simulink model "target_transmit_singleThreshold_MFB"  (R2015a)
settings: Solver=FixedStepDiscrete  StartTime=0  StopTime=inf  RelTol=1e-3
model workspace (MAT data in the model file):
  dt = 0.1
undefined symbols (not defined in the file or in its folder): gray, IsPositionTracked, IsSkeletonTracked, jet, JointDepthIndices, JointImageIndices, JointTrackingState, JointWorldCoordinates, none, PositionDepthIndices, PositionImageIndices, PositionWorldCoordinates, SegmentationData, SkeletonTrackingID, videoinput
libraries: visionsinks x5, visiontextngfix x3, embdlinuxlib x2, visionconversions x1, dspvision x1, imaqlib x1, sldrtlib x1
settings Model: PauseTimes=89  ExtModeTrigDuration=100  Creator=sbiagion  LastModifiedBy=sbiagion
settings DataIOCC: SaveFormat=StructureWithTime
settings OptimizationCC: OptimizeModelRefInitCode=on  LifeSpan=1
settings DebuggingCC: UnderspecifiedInitializationDetection=Classic  MergeDetectMultiDrivingBlocksExec=none
settings HardwareCC: ProdLargestAtomicInteger=Long  ProdLargestAtomicFloat=Double  ProdEndianess=LittleEndian  ProdHWDeviceType=ARM Compatible->ARM Cortex
settings RTWCC: SystemTargetFile=realtime.tlc  GenerateMakefile=off  TemplateMakefile=realtime.tmf  Description=Run on Target Hardware  RTWVerbose=off
settings STFCustomTargetCC: CodeReplacementLibrary=C89/C90 (ANSI)
settings ERTTargetCC: CodeReplacementLibrary=C89/C90 (ANSI)  CombineOutputUpdateFcns=off  ExtModeMexArgs='172.28.64.170' 0 17725  ERTSrcFileBannerTemplate=realtime_code_template.cgt  ERTHdrFileBannerTemplate=realtime_code_template.cgt  ERTDataSrcFileTemplate=realtime_code_template.cgt  ERTDataHdrFileTemplate=realtime_code_template.cgt  ERTCustomFileTemplate=realtime_file_process.tlc

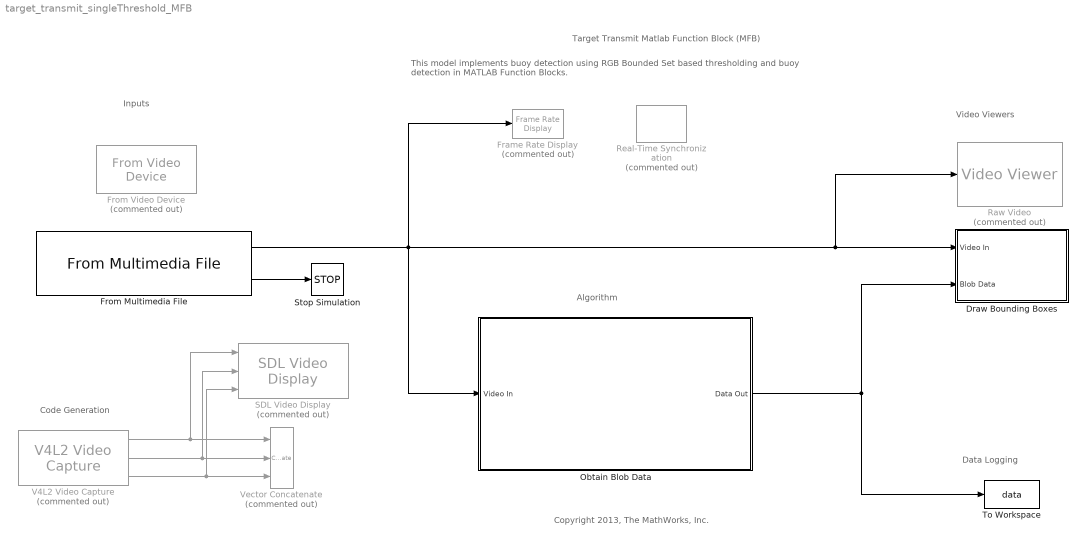
== system target_transmit_singleThreshold_MFB ==
  note: Copyright 2013, The MathWorks, Inc.
  note: Data Logging
  note: Algorithm
  note: Video Viewers
  note: Inputs
  note: Code Generation
  note: This model implements buoy detection using RGB Bounded Set based thresholding
      | and buoy detection in MATLAB Function Blocks.
  note: Target Transmit Matlab Function Block (MFB)
  Draw Bounding Boxes : Subsystem
  Frame Rate Display : visionsinks/Frame Rate Display  Commented=on  UpdateRate=10
  From Multimedia File : dspvision/From Multimedia File  inputFilename=..\..\media\rawVideo_640x480.avi  loop=on  numPlays=1  outputStreams=Video only  videoDataType=uint8  audioDataType=int16  inheritSampleTime=on  userDefinedSampleTime=0.1  noAudioOutput=off  isIntensityVideo=off  fourcc=RGB  colorVideoFormat=One multidimensional signal  outputEOF=on  dataOrg=Column-major  audioFrameSize=1024  computeAudioFrameSize=off  outSamplingMode=Sample based
  From Video Device : imaqlib/From Video Device  Commented=on  DeviceMenu=(none)  Device=winvideo 1 (Microsoft LifeCam Cinema)  ObjConstructor=videoinput('winvideo', 1)  VideoFormatMenu=(none)  VideoFormat=MJPG_640x480  VideoSource=input1  ROIPosition=[0 0 480 640]  EnableHWTrigger=off  TriggerConfiguration=none/none  SampleTime=0.1  OutputPortsMode=One multidimensional signal  DataType=single  CanDoHWTrigger=no  ReturnedColorSpace=rgb  BlockHandle=2792.0001  ROIWidth=640  ROIHeight=480  ROIColumn=0  ROIRow=0  EngXMLPath=C:\Program Files\MATLAB\R2015a\toolbox\imaq\imaq\private  DevXMLPath=C:\Program Files\MATLAB\R2015a\toolbox\imaq\imaqadaptors\win64  EngLibPath=C:\Program Files\MATLAB\R2015a\toolbox\imaq\imaqblks\imaqmex\win64  ColorSpace=rgb  BayerSensorAlignment=grbg  AllMetadata=IsPositionTracked;IsSkeletonTracked;JointDepthIndices;JointImageIndices;JointTrackingState;JointWorldCoordinates;PositionDepthIndices;PositionImageIndices;PositionWorldCoordinates;SegmentationData;SkeletonTrackingID
  Obtain Blob Data : Subsystem  VariantControl=boundedVariant
  "Raw Video " : visionsinks/Video Viewer  Commented=on  inputType=Obsolete7b  imagePorts=One multidimensional signal  useColorMap=off  colormapValue=gray(256)  specRange=off  minInputVal=0  maxInputVal=255  FigPos=[1096 875 817 565]  AxisZoom=on  trueSizedOnce=off  OpenAtMdlStart=on  DefaultConfigurationName=vipscopes.VideoViewerScopeCfg
  Real-Time Synchronization : sldrtlib/Real-Time Synchronization  Commented=on  SampleTime=0.1  MaxMissedTicks=1e9  ShowMissedTicks=off  YieldWhenWaiting=off
  SDL Video Display : embdlinuxlib/SDL Video Display  Commented=on  pixelFormat=RGB  pixelOrder=Planar  rowMajor=on  blockPlatform=BeagleBoard
  Stop Simulation : Stop
  To Workspace : ToWorkspace  VariableName=data  SaveFormat=Timeseries  SampleTime=-1
  V4L2 Video Capture : embdlinuxlib/V4L2 Video Capture  Commented=on  m_devName='/dev/video0'  roi=[0, 0, 640, 480]  imSizeSelection=640x480  imSize=[640, 480]  pixelFormat=RGB  pixelOrder=Planar  sampleTime=1/30  simOutput=Colorbars  blockPlatform=BeagleBoard
  Vector Concatenate : Concatenate  Commented=on  NumInputs=3  Mode=Multidimensional array  ConcatenateDimension=3
  wires:
  From Multimedia File/2 -> Stop Simulation/1
  V4L2 Video Capture/1 -> SDL Video Display/1, Vector Concatenate/1
  V4L2 Video Capture/2 -> SDL Video Display/2, Vector Concatenate/2
  V4L2 Video Capture/3 -> SDL Video Display/3, Vector Concatenate/3
  Obtain Blob Data/1(Data Out) -> Draw Bounding Boxes/2(Blob Data), To Workspace/1
  From Multimedia File/1 -> Obtain Blob Data/1(Video In), Frame Rate Display/1, Draw Bounding Boxes/1(Video In), "Raw Video "/1

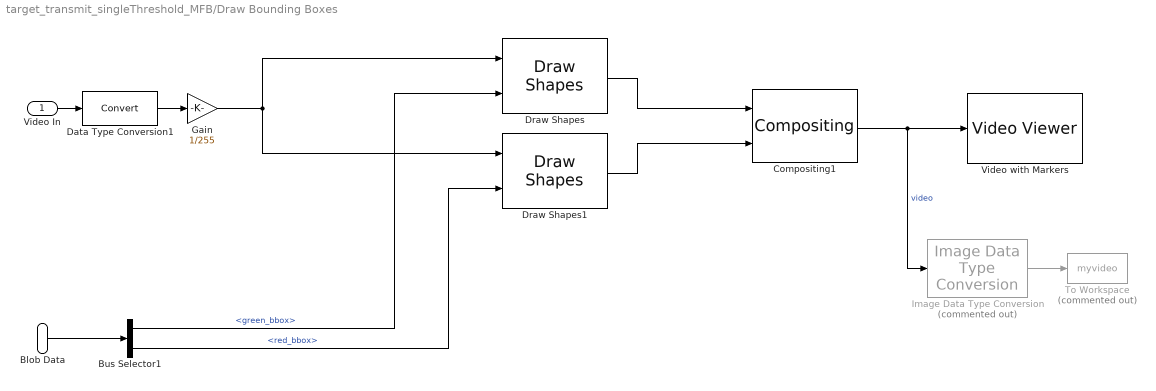
== system target_transmit_singleThreshold_MFB/Draw Bounding Boxes ==
  Video In : Inport
  Blob Data : Inport  Port=2
  Bus Selector1 : BusSelector  OutputSignals=green_bbox,red_bbox
  Compositing1 : visiontextngfix/Compositing  operation=Blend  bFacSrc=Specify via dialog  mFacSrc=Specify via dialog  bFactor=0.75  mFactor=1  source=Specify via dialog  coordinates=[1 1]  prodOutputMode=Binary point scaling  prodOutputWordLength=32  prodOutputFracLength=10  roundingMode=Floor  overflowMode=off
  Data Type Conversion1 : DataTypeConversion
  Draw Shapes : visiontextngfix/Draw Shapes  shape=Rectangles  fill=on  lineWidth=1  fillClrSource=Specify via dialog  display=User-specified value  intensity=200  color=[0 255 0]  opacity=0.5  viewport=Entire image  antialiasing=off  inType=Obsolete  imagePorts=One multidimensional signal  prodOutputMode=Binary point scaling  prodOutputWordLength=32  prodOutputFracLength=14  memoryMode=Specify word length  memoryWordLength=16  memoryFracLength=14  roundingMode=Floor  overflowMode=off
  Draw Shapes1 : visiontextngfix/Draw Shapes  shape=Rectangles  fill=on  lineWidth=1  fillClrSource=Specify via dialog  display=User-specified value  intensity=200  color=[255 0 0]  opacity=0.5  viewport=Entire image  antialiasing=off  inType=Obsolete  imagePorts=One multidimensional signal  prodOutputMode=Binary point scaling  prodOutputWordLength=32  prodOutputFracLength=14  memoryMode=Specify word length  memoryWordLength=16  memoryFracLength=14  roundingMode=Floor  overflowMode=off
  Gain : Gain  Gain=1/255
  Image Data Type Conversion : visionconversions/Image Data Type Conversion  Commented=on  outDT=uint8  isSigned=on  wordLen=16  numFracBits=0
  To Workspace : ToWorkspace  Commented=on  VariableName=myvideo  SaveFormat=Timeseries  SampleTime=-1
  Video with Markers : visionsinks/Video Viewer  inputType=Obsolete7b  imagePorts=One multidimensional signal  useColorMap=off  colormapValue=gray(256)  specRange=off  minInputVal=0  maxInputVal=255  FigPos=[791 911 843 656]  AxisZoom=on  trueSizedOnce=off  OpenAtMdlStart=on  DefaultConfigurationName=vipscopes.VideoViewerScopeCfg
  wires:
  Gain/1 -> Draw Shapes/1, Draw Shapes1/1
  Data Type Conversion1/1 -> Gain/1
  Draw Shapes1/1 -> Compositing1/2
  Draw Shapes/1 -> Compositing1/1
  Bus Selector1/1 -> Draw Shapes/2  "<green_bbox>"
  Blob Data/1 -> Bus Selector1/1
  Video In/1 -> Data Type Conversion1/1
  Compositing1/1 -> Image Data Type Conversion/1, Video with Markers/1  "video"
  Bus Selector1/2 -> Draw Shapes1/2  "<red_bbox>"
  Image Data Type Conversion/1 -> To Workspace/1

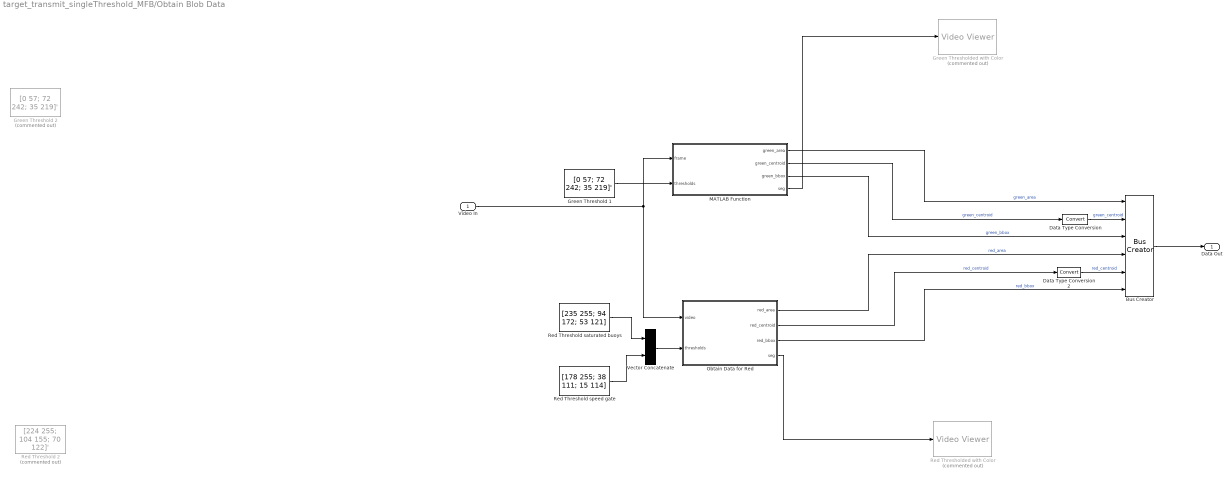
== system target_transmit_singleThreshold_MFB/Obtain Blob Data ==
  Video In : Inport
  Bus Creator : BusCreator  Inputs=6
  Data Type Conversion : DataTypeConversion
  Data Type Conversion2 : DataTypeConversion
  Green Threshold 1 : Constant  Value=[0 57; 72 242; 35 219]'  OutDataTypeStr=uint8
  Green Threshold 2 : Constant  Commented=on  Value=[0 57; 72 242; 35 219]'  OutDataTypeStr=uint8
  Green Thresholded with Color : visionsinks/Video Viewer  Commented=on  inputType=Obsolete7b  imagePorts=One multidimensional signal  useColorMap=off  colormapValue=gray(256)  specRange=off  minInputVal=0  maxInputVal=255  FigPos=[531 770 672 453]  AxisZoom=on  trueSizedOnce=off  OpenAtMdlStart=on  DefaultConfigurationName=vipscopes.VideoViewerScopeCfg
  MATLAB Function : MATLAB Function  TreatAsAtomicUnit=on
  Obtain Data for Red : MATLAB Function  TreatAsAtomicUnit=on
  Red Threshold 2 : Constant  Commented=on  Value=[224 255; 104 155; 70 122]'  OutDataTypeStr=uint8
  Red Threshold saturated buoys : Constant  Value=[235 255; 94 172; 53 121]  OutDataTypeStr=uint8
  Red Threshold speed gate : Constant  Value=[178 255; 38 111; 15 114]  OutDataTypeStr=uint8
  Red Thresholded with Color : visionsinks/Video Viewer  Commented=on  inputType=Obsolete7b  imagePorts=One multidimensional signal  useColorMap=off  colormapValue=jet(256)  specRange=off  minInputVal=0  maxInputVal=255  FigPos=[555 1047 410 300]  AxisZoom=on  trueSizedOnce=off  OpenAtMdlStart=on  DefaultConfigurationName=vipscopes.VideoViewerScopeCfg
  Vector Concatenate : Concatenate  Mode=Multidimensional array
  Data Out : Outport
  wires:
  Green Threshold 1/1 -> MATLAB Function/2(thresholds)
  MATLAB Function/3(green_bbox) -> Bus Creator/3  "green_bbox"
  MATLAB Function/2(green_centroid) -> Data Type Conversion/1  "green_centroid"
  MATLAB Function/1(green_area) -> Bus Creator/1  "green_area"
  Obtain Data for Red/1(red_area) -> Bus Creator/4  "red_area"
  Obtain Data for Red/2(red_centroid) -> Data Type Conversion2/1  "red_centroid"
  Bus Creator/1 -> Data Out/1
  Data Type Conversion/1 -> Bus Creator/2  "green_centroid"
  Data Type Conversion2/1 -> Bus Creator/5  "red_centroid"
  Obtain Data for Red/3(red_bbox) -> Bus Creator/6  "red_bbox"
  Vector Concatenate/1 -> Obtain Data for Red/2(thresholds)
  Red Threshold speed gate/1 -> Vector Concatenate/2
  Red Threshold saturated buoys/1 -> Vector Concatenate/1
  Video In/1 -> MATLAB Function/1(frame), Obtain Data for Red/1(video)
  Obtain Data for Red/4(seg) -> Red Thresholded with Color/1
  MATLAB Function/4(seg) -> Green Thresholded with Color/1

== matlab function target_transmit_singleThreshold_MFB/Obtain Blob Data/MATLAB Function ==
  data: frame input; green_area output; thresholds input; green_centroid output; green_bbox output; seg output
function [green_area, green_centroid, green_bbox,seg] = test_thresholdingMatlab(frame,thresholds)
%#codegen

%% initialization
% initialize blob analysis object
blobAnalysisObject = vision.BlobAnalysis('AreaOutputPort',true,'BoundingBoxOutputPort',true,'MinimumBlobArea',40,'MaximumCount',4);

%% algorithm
% segment the RGB frame to obtain the segmented black and white image
bw = thresholdImage(frame,thresholds);

% perform blob detection
[blob_area,blob_centroid,blob_bbox] = step(blobAnalysisObject,bw);
nblobs = length(blob_area);

%% extra visualization
seg = bw;

%% output data
% initialize output data so that is fixed
green_area = -ones(4,1);
green_centroid = -ones(4,2);
green_bbox = -ones(4,4);

green_area(1:nblobs) = blob_area;
green_centroid(1:nblobs,:) = blob_centroid;
green_bbox(1:nblobs,:) = blob_bbox;

function bw = thresholdImage(img,thresholds)
    bw = false(480,640);
    nt = size(thresholds,2)/3; % bad for mfb
%     nt = 1; % good for mfbe
    for i = 1:nt
    bw = bw | logical(... % red threshold
            img(:,:,1)>=thresholds(1,3*i-2) & ...
            img(:,:,1)<=thresholds(2,3*i-2)  & ...
            ... % green threshold
            img(:,:,2)>=thresholds(1,3*i-1) & ...           
            img(:,:,2)<=thresholds(2,3*i-1)  & ...  
            ... % blue threshold
            img(:,:,3)>=thresholds(1,3*i) & ... 
            img(:,:,3)<=thresholds(2,3*i));
    end

== matlab function target_transmit_singleThreshold_MFB/Obtain Blob Data/Obtain Data for Red ==
  data: video input; red_area output; red_centroid output size=[4 2]; thresholds input; red_bbox output size=[4 4]; seg output
function [red_area,red_centroid,red_bbox,seg]  = fcn(video,thresholds)
%#codegen

%% initialization
hBlob = vision.BlobAnalysis('AreaOutputPort',true,'BoundingBoxOutputPort',true,'MinimumBlobArea',20,'MaximumCount',4);  
bw = false(480,640);

% segment the RGB frame to obtain the segmented black and white image
nthresholds = 2;
for idx = 1:nthresholds
    bw = bw | logical(... % red threshold
        video(:,:,1)>=thresholds(3*idx-2,1) & ...
        video(:,:,1)<=thresholds(3*idx-2,2)  & ...
        ... % green threshold
        video(:,:,2)>=thresholds(3*idx-1,1) & ...           
        video(:,:,2)<=thresholds(3*idx-1,2)  & ...  
        ... % blue threshold
        video(:,:,3)>=thresholds(3*idx,1) & ... 
        video(:,:,3)<=thresholds(3*idx,2));      
end
        
% overlay color onto thresholded bw image
% can be used to clean up noise easily
% comment out if unnecessary
colorseg = uint8(repmat(bw,[1,1,3]).*double(video));

% % close operation
bw = bwmorph(bw,'close');
        
% perform blob detection
[blob_area,blob_centroid,blob_bbox] = step(hBlob,bw);
nblobs = length(blob_area);

% output red data
red_area = -ones(4,1);
red_centroid = -ones(4,2);
red_bbox = -ones(4,4);

red_area(1:nblobs) = blob_area;
red_centroid(1:nblobs,:) = blob_centroid;
red_bbox(1:nblobs,:) = blob_bbox;

%%
seg = colorseg;
